simulink model "Calibration"  (R2018b)
settings: Solver=VariableStepAuto  StartTime=0.0  StopTime=10.0  RelTol=1e-3
settings Model: Creator=M18001  LastModifiedBy=M18001

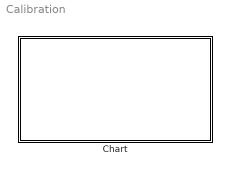
== system Calibration ==
  Chart : Stateflow chart  TreatAsAtomicUnit=on

== stateflow chart Calibration/Chart ==
  note: 1.Init
      | R = 0.001;
      | v = v = zeros(9,1);
      | if sensor == acc
      | P = diag([10,10,10,0,0,0,1,1,1]);
      | elseif sensor == mag
      | P = diag([10,10,10,1,1,1,1,1,1]);
      | end
      |
      | 2. Step
      | [next_v, next_P] = ellipsoid_fit_step(x,y,z,v,P,R)
      | where x,y,z is raw mag data
      |
      | 3. Solve
      | [mat, bias, u, radii] = ellipsoid_fit_solve(v)
      | where mat is rotation mateix. mat and bias will be used for sensor calibration
      |
      | 4. Calculate Error
      | for all mag data (x,z,y)
      | fit_val = u(1) *x.*x + u(2) * y.*y + u(3) * z.*z + ...
      | 2*u(4) *x.*y + 2*u(5)*x.*z + 2*u(6) * y.*z + ...
      | 2*u(7) *x + 2*u(8)*y + 2*u(9) * z;
      | isovalue = mean(fit_val);
      | error = 1-isovalue
  data: x function_input; y function_input; z function_input; v function_input; P function_input; R function_input; next_v function_output; next_P function_output; v function_input; mat function_output; bias function_output; u function_output; radii function_output
  function [next_v, next_P] = ellipsoid_fit_step(x,y,z,v,P,R):
    | function [next_v, next_P] = ellipsoid_fit_step(x,y,z,v,P,R)
    | 
    | H = [x^2, y^2, z^2, 2*x*y, 2*x*z, 2*y*z, 2*x, 2*y, 2*z];
    | 
    | Y = 1 - H*v;
    | % S(k) = H(k)*P(k|k-1)*H(k)' + R(k)
    | S = H*P*H' + R;
    | % K(k) = P(k|k-1)*H(k)'*S(k)^-1
    | K = P*H'/S; 
    | % X(k|k) = X(k|k-1) + K(k)*Y(k)
    | v = v + K*Y;
    | % P(k|k) = P(k|k-1) - K(k)*H(k)*P(k|k-1);
    | P = P - K*H*P;
    | %     P = (eye(9)-K*H)*P*(eye(9)-K*H)'+K*R*K';
    | 
    | next_v = v;
    | next_P = P;
    | 
    | end
  function [mat, bias, u, radii] = ellipsoid_fit_solve(v):
    | function [mat, bias, u, radii] = ellipsoid_fit_solve(v)
    | 
    | A = [ v(1) v(4) v(5) v(7); v(4) v(2) v(6) v(8); v(5) v(6) v(3) v(9); v(7) v(8) v(9) -1 ];
    | ofs=-A(1:3,1:3)\[v(7);v(8);v(9)]; % offset is center of ellipsoid
    | Tmtx=eye(4); Tmtx(4,1:3)=ofs'; AT=Tmtx*A*Tmtx'; % ellipsoid translated to (0,0,0)
    | [evecs ev]=eig(AT(1:3,1:3)/-AT(4,4)); % eigenvectors (rotation) and eigenvalues (gain)
    | gain=sqrt(1./diag(ev)); % gain is radius of the ellipsoid
    | 
    | g_mat = diag(1./gain);
    | % g_mat = diag(sqrt(diag(ev)));
    | % g_mat will rotate axis, so we need rotate axis back
    | trans_mat = evecs*g_mat*pinv(evecs);
    | % main the norm of input data
    | trans_mat = trans_mat'/norm(trans_mat);
    | 
    | bias = ofs;
    | mat = trans_mat;
    | u = v;
    | radii = gain;
    | 
    | end
